simulink model "power_wind"  (R2014b)
settings: Solver=ode23tb  StartTime=0.0  StopTime=20  MaxStep=1/60  RelTol=1e-4  AbsTol=1e-3
InitFcn:
  | xInitial = init_power_wind_ig;
undefined symbols (not defined in the file): D1, D11, Delta
libraries: powerlib_meascontrol x45, powerlib x29, DRlib x3, factslib x1
(part 2 of 4)

== system power_wind/Wind Farm/Wind Turbine Protections/Protection System1/Decoding ==
  Code : Inport
  Constant : Constant  Value=pow2(0:-1:-9)
  Constant6 : Constant  Value=2
  Math Function : Math  Operator=rem  SaturateOnIntegerOverflow=on
  Product : Product  SaturateOnIntegerOverflow=on  InputSameDT=on  OutDataTypeStr=Inherit: Same as first input
  Rounding Function : Rounding
  Out : Outport
  wires:
  Math Function/1 -> Out/1
  Rounding Function/1 -> Math Function/1
  Constant6/1 -> Math Function/2
  Product/1 -> Rounding Function/1
  Code/1 -> Product/1
  Constant/1 -> Product/2

== system power_wind/Wind Farm/Wind Turbine Protections/Protection System1/Encoding ==
  In1 : Inport
  In2 : Inport  Port=2
  In3 : Inport  Port=3
  In4 : Inport  Port=4
  In5 : Inport  Port=5
  In6 : Inport  Port=6
  In7 : Inport  Port=7
  In8 : Inport  Port=8
  In9 : Inport  Port=9
  In10 : Inport  Port=10
  Constant12 : Constant  Value=pow2(0:1:9)
  Data Type Conversion : DataTypeConversion  SaturateOnIntegerOverflow=on  RndMeth=Zero
  Mux : Mux  Inputs=10
  Product : Product  SaturateOnIntegerOverflow=on  InputSameDT=on  OutDataTypeStr=Inherit: Same as first input
  Sum : Sum  Inputs=1  SaturateOnIntegerOverflow=on  InputSameDT=on  OutDataTypeStr=Inherit: Same as first input
  Code : Outport
  wires:
  Sum/1 -> Code/1
  Constant12/1 -> Product/2
  Product/1 -> Sum/1
  In1/1 -> Mux/1
  In10/1 -> Mux/10
  In9/1 -> Mux/9
  In8/1 -> Mux/8
  In7/1 -> Mux/7
  In6/1 -> Mux/6
  In5/1 -> Mux/5
  In4/1 -> Mux/4
  In3/1 -> Mux/3
  In2/1 -> Mux/2
  Mux/1 -> Data Type Conversion/1
  Data Type Conversion/1 -> Product/1

== system power_wind/Wind Farm/Wind Turbine Protections/Protection System1/Under//Over Speed Protection ==
  Speed : Inport  PortDimensions=1
  On Delay : powerlib_meascontrol/Logic/On Delay  DelayType=On delay  delay=Delay_Speed  ic=0  Ts=0
  On Delay1 : powerlib_meascontrol/Logic/On Delay  DelayType=On delay  delay=Delay_Speed  ic=0  Ts=0
  Relational Operator1 : RelationalOperator  Operator=>
  Relational Operator3 : RelationalOperator  Operator=<
  V1 max1 : Constant  Value=Min_Speed
  V1 max3 : Constant  Value=Max_Speed
  MinSpeed : Outport
  MaxSpeed : Outport  Port=2
  wires:
  On Delay1/1 -> MaxSpeed/1
  On Delay/1 -> MinSpeed/1
  Speed/1 -> Relational Operator1/1, Relational Operator3/1
  V1 max3/1 -> Relational Operator1/2
  V1 max1/1 -> Relational Operator3/2
  Relational Operator1/1 -> On Delay1/1
  Relational Operator3/1 -> On Delay/1

== system power_wind/Wind Farm/Wind Turbine Protections/Protection System2/AC Current Protection ==
  abc : Inport  PortDimensions=3
  Complex to Magnitude-Angle1 : ComplexToMagnitudeAngle  Output=Magnitude
  Current Measurement : Subsystem
  MinMax : MinMax  Function=max  ZeroCross=off  SaturateOnIntegerOverflow=on  InputSameDT=on
  Mux : Mux  Inputs=3
  On Delay : powerlib_meascontrol/Logic/On Delay  DelayType=On delay  delay=Delay_I1  ic=0  Ts=0
  On Delay1 : powerlib_meascontrol/Logic/On Delay  DelayType=On delay  delay=Delay_I2_I1  ic=0  Ts=0
  Relational Operator10 : RelationalOperator  Operator=>
  Relational Operator6 : RelationalOperator  Operator=>
  Relational Operator8 : RelationalOperator  Operator=>
  Selector : Selector  InputPortWidth=3
  Selector1 : Selector  InputPortWidth=3  Indices=2
  Selector2 : Selector  InputPortWidth=3  Indices=3
  V0/V1 max3 : Constant  Value=Max_I1
  V1 max : Constant  Value=Max_I2_I1
  V1 max2 : Constant  Value=Max_Iinst
  MaxIinst : Outport
  MaxI1 : Outport  Port=2
  MaxI2I1 : Outport  Port=3
  wires:
  abc/1 -> Current Measurement/1(abc), Selector/1, Selector1/1, Selector2/1
  Current Measurement/1(I1) -> Relational Operator6/1
  V0/V1 max3/1 -> Relational Operator6/2
  V1 max/1 -> Relational Operator8/2
  Current Measurement/2(I2/I1) -> Relational Operator8/1
  Relational Operator6/1 -> On Delay/1
  Relational Operator8/1 -> On Delay1/1
  On Delay/1 -> MaxI1/1
  On Delay1/1 -> MaxI2I1/1
  Relational Operator10/1 -> MaxIinst/1
  V1 max2/1 -> Relational Operator10/2
  Selector/1 -> Mux/1
  Selector2/1 -> Mux/3
  Selector1/1 -> Mux/2
  Mux/1 -> Complex to Magnitude-Angle1/1
  Complex to Magnitude-Angle1/1 -> MinMax/1
  MinMax/1 -> Relational Operator10/1

== system power_wind/Wind Farm/Wind Turbine Protections/Protection System2/AC Voltage Protection ==
  abc : Inport  PortDimensions=3
  On Delay : powerlib_meascontrol/Logic/On Delay  DelayType=On delay  delay=Delay_V1  ic=0  Ts=0
  On Delay1 : powerlib_meascontrol/Logic/On Delay  DelayType=On delay  delay=Delay_V1  ic=0  Ts=0
  On Delay2 : powerlib_meascontrol/Logic/On Delay  DelayType=On delay  delay=Delay_V2_V1  ic=0  Ts=0
  On Delay3 : powerlib_meascontrol/Logic/On Delay  DelayType=On delay  delay=Delay_V2_V1  ic=0  Ts=0
  Relational Operator6 : RelationalOperator  Operator=>
  Relational Operator7 : RelationalOperator  Operator=<
  Relational Operator8 : RelationalOperator  Operator=>
  Relational Operator9 : RelationalOperator  Operator=>
  V0/V1 max3 : Constant  Value=Max_V1
  V0/V1 max4 : Constant  Value=Min_V1
  V1 max : Constant  Value=Max_V2_V1
  V1 max1 : Constant  Value=Max_V0_V1
  Voltage Measurement : Subsystem
  MinV1 : Outport
  MaxV1 : Outport  Port=2
  MaxV2V1 : Outport  Port=3
  MaxV0V1 : Outport  Port=4
  wires:
  On Delay3/1 -> MaxV0V1/1
  On Delay2/1 -> MaxV2V1/1
  On Delay/1 -> MinV1/1
  On Delay1/1 -> MaxV1/1
  Relational Operator9/1 -> On Delay3/1
  Relational Operator8/1 -> On Delay2/1
  Relational Operator7/1 -> On Delay/1
  Relational Operator6/1 -> On Delay1/1
  Voltage Measurement/3(V0/V1) -> Relational Operator9/1
  V1 max1/1 -> Relational Operator9/2
  Voltage Measurement/2(V2/V1) -> Relational Operator8/1
  V1 max/1 -> Relational Operator8/2
  V0/V1 max4/1 -> Relational Operator7/2
  V0/V1 max3/1 -> Relational Operator6/2
  Voltage Measurement/1(V1) -> Relational Operator7/1, Relational Operator6/1
  abc/1 -> Voltage Measurement/1(abc)

== system power_wind/Wind Farm/Wind Turbine Protections/Protection System2/DC Voltage Protection ==
  Vdc : Inport
  On Delay : powerlib_meascontrol/Logic/On Delay  DelayType=On delay  delay=Delay_Vdc  ic=0  Ts=0
  Relational Operator1 : RelationalOperator  Operator=>
  V1 max3 : Constant  Value=Max_Vdc
  MaxVdc : Outport
  wires:
  Vdc/1 -> Relational Operator1/1
  V1 max3/1 -> Relational Operator1/2
  Relational Operator1/1 -> On Delay/1
  On Delay/1 -> MaxVdc/1

== system power_wind/Wind Farm/Wind Turbine Protections/Protection System2/Decoding ==
  Code : Inport
  Constant : Constant  Value=pow2(0:-1:-9)
  Constant6 : Constant  Value=2
  Math Function : Math  Operator=rem  SaturateOnIntegerOverflow=on
  Product : Product  SaturateOnIntegerOverflow=on  InputSameDT=on  OutDataTypeStr=Inherit: Same as first input
  Rounding Function : Rounding
  Out : Outport
  wires:
  Constant/1 -> Product/2
  Code/1 -> Product/1
  Product/1 -> Rounding Function/1
  Constant6/1 -> Math Function/2
  Rounding Function/1 -> Math Function/1
  Math Function/1 -> Out/1

== system power_wind/Wind Farm/Wind Turbine Protections/Protection System2/Encoding ==
  In1 : Inport
  In2 : Inport  Port=2
  In3 : Inport  Port=3
  In4 : Inport  Port=4
  In5 : Inport  Port=5
  In6 : Inport  Port=6
  In7 : Inport  Port=7
  In8 : Inport  Port=8
  In9 : Inport  Port=9
  In10 : Inport  Port=10
  Constant12 : Constant  Value=pow2(0:1:9)
  Data Type Conversion : DataTypeConversion  SaturateOnIntegerOverflow=on  RndMeth=Zero
  Mux : Mux  Inputs=10
  Product : Product  SaturateOnIntegerOverflow=on  InputSameDT=on  OutDataTypeStr=Inherit: Same as first input
  Sum : Sum  Inputs=1  SaturateOnIntegerOverflow=on  InputSameDT=on  OutDataTypeStr=Inherit: Same as first input
  Code : Outport
  wires:
  Data Type Conversion/1 -> Product/1
  Mux/1 -> Data Type Conversion/1
  In2/1 -> Mux/2
  In3/1 -> Mux/3
  In4/1 -> Mux/4
  In5/1 -> Mux/5
  In6/1 -> Mux/6
  In7/1 -> Mux/7
  In8/1 -> Mux/8
  In9/1 -> Mux/9
  In10/1 -> Mux/10
  In1/1 -> Mux/1
  Product/1 -> Sum/1
  Constant12/1 -> Product/2
  Sum/1 -> Code/1

== system power_wind/Wind Farm/Wind Turbine Protections/Protection System2/Under//Over Speed Protection ==
  Speed : Inport  PortDimensions=1
  On Delay : powerlib_meascontrol/Logic/On Delay  DelayType=On delay  delay=Delay_Speed  ic=0  Ts=0
  On Delay1 : powerlib_meascontrol/Logic/On Delay  DelayType=On delay  delay=Delay_Speed  ic=0  Ts=0
  Relational Operator1 : RelationalOperator  Operator=>
  Relational Operator3 : RelationalOperator  Operator=<
  V1 max1 : Constant  Value=Min_Speed
  V1 max3 : Constant  Value=Max_Speed
  MinSpeed : Outport
  MaxSpeed : Outport  Port=2
  wires:
  Relational Operator3/1 -> On Delay/1
  Relational Operator1/1 -> On Delay1/1
  V1 max1/1 -> Relational Operator3/2
  V1 max3/1 -> Relational Operator1/2
  Speed/1 -> Relational Operator3/1, Relational Operator1/1
  On Delay/1 -> MinSpeed/1
  On Delay1/1 -> MaxSpeed/1

== system power_wind/Wind Farm/Wind Turbine Protections/Protection System3/AC Current Protection ==
  abc : Inport  PortDimensions=3
  Complex to Magnitude-Angle1 : ComplexToMagnitudeAngle  Output=Magnitude
  Current Measurement : Subsystem
  MinMax : MinMax  Function=max  ZeroCross=off  SaturateOnIntegerOverflow=on  InputSameDT=on
  Mux : Mux  Inputs=3
  On Delay : powerlib_meascontrol/Logic/On Delay  DelayType=On delay  delay=Delay_I1  ic=0  Ts=0
  On Delay1 : powerlib_meascontrol/Logic/On Delay  DelayType=On delay  delay=Delay_I2_I1  ic=0  Ts=0
  Relational Operator10 : RelationalOperator  Operator=>
  Relational Operator6 : RelationalOperator  Operator=>
  Relational Operator8 : RelationalOperator  Operator=>
  Selector : Selector  InputPortWidth=3
  Selector1 : Selector  InputPortWidth=3  Indices=2
  Selector2 : Selector  InputPortWidth=3  Indices=3
  V0/V1 max3 : Constant  Value=Max_I1
  V1 max : Constant  Value=Max_I2_I1
  V1 max2 : Constant  Value=Max_Iinst
  MaxIinst : Outport
  MaxI1 : Outport  Port=2
  MaxI2I1 : Outport  Port=3
  wires:
  MinMax/1 -> Relational Operator10/1
  Complex to Magnitude-Angle1/1 -> MinMax/1
  Mux/1 -> Complex to Magnitude-Angle1/1
  Selector1/1 -> Mux/2
  Selector2/1 -> Mux/3
  Selector/1 -> Mux/1
  V1 max2/1 -> Relational Operator10/2
  Relational Operator10/1 -> MaxIinst/1
  On Delay1/1 -> MaxI2I1/1
  On Delay/1 -> MaxI1/1
  Relational Operator8/1 -> On Delay1/1
  Relational Operator6/1 -> On Delay/1
  Current Measurement/2(I2/I1) -> Relational Operator8/1
  V1 max/1 -> Relational Operator8/2
  V0/V1 max3/1 -> Relational Operator6/2
  Current Measurement/1(I1) -> Relational Operator6/1
  abc/1 -> Selector2/1, Selector1/1, Selector/1, Current Measurement/1(abc)

== system power_wind/Wind Farm/Wind Turbine Protections/Protection System3/AC Voltage Protection ==
  abc : Inport  PortDimensions=3
  On Delay : powerlib_meascontrol/Logic/On Delay  DelayType=On delay  delay=Delay_V1  ic=0  Ts=0
  On Delay1 : powerlib_meascontrol/Logic/On Delay  DelayType=On delay  delay=Delay_V1  ic=0  Ts=0
  On Delay2 : powerlib_meascontrol/Logic/On Delay  DelayType=On delay  delay=Delay_V2_V1  ic=0  Ts=0
  On Delay3 : powerlib_meascontrol/Logic/On Delay  DelayType=On delay  delay=Delay_V2_V1  ic=0  Ts=0
  Relational Operator6 : RelationalOperator  Operator=>
  Relational Operator7 : RelationalOperator  Operator=<
  Relational Operator8 : RelationalOperator  Operator=>
  Relational Operator9 : RelationalOperator  Operator=>
  V0/V1 max3 : Constant  Value=Max_V1
  V0/V1 max4 : Constant  Value=Min_V1
  V1 max : Constant  Value=Max_V2_V1
  V1 max1 : Constant  Value=Max_V0_V1
  Voltage Measurement : Subsystem
  MinV1 : Outport
  MaxV1 : Outport  Port=2
  MaxV2V1 : Outport  Port=3
  MaxV0V1 : Outport  Port=4
  wires:
  abc/1 -> Voltage Measurement/1(abc)
  Voltage Measurement/1(V1) -> Relational Operator6/1, Relational Operator7/1
  V0/V1 max3/1 -> Relational Operator6/2
  V0/V1 max4/1 -> Relational Operator7/2
  V1 max/1 -> Relational Operator8/2
  Voltage Measurement/2(V2/V1) -> Relational Operator8/1
  V1 max1/1 -> Relational Operator9/2
  Voltage Measurement/3(V0/V1) -> Relational Operator9/1
  Relational Operator6/1 -> On Delay1/1
  Relational Operator7/1 -> On Delay/1
  Relational Operator8/1 -> On Delay2/1
  Relational Operator9/1 -> On Delay3/1
  On Delay1/1 -> MaxV1/1
  On Delay/1 -> MinV1/1
  On Delay2/1 -> MaxV2V1/1
  On Delay3/1 -> MaxV0V1/1

== system power_wind/Wind Farm/Wind Turbine Protections/Protection System3/DC Voltage Protection ==
  Vdc : Inport
  On Delay : powerlib_meascontrol/Logic/On Delay  DelayType=On delay  delay=Delay_Vdc  ic=0  Ts=0
  Relational Operator1 : RelationalOperator  Operator=>
  V1 max3 : Constant  Value=Max_Vdc
  MaxVdc : Outport
  wires:
  On Delay/1 -> MaxVdc/1
  Relational Operator1/1 -> On Delay/1
  V1 max3/1 -> Relational Operator1/2
  Vdc/1 -> Relational Operator1/1

== system power_wind/Wind Farm/Wind Turbine Protections/Protection System3/Decoding ==
  Code : Inport
  Constant : Constant  Value=pow2(0:-1:-9)
  Constant6 : Constant  Value=2
  Math Function : Math  Operator=rem  SaturateOnIntegerOverflow=on
  Product : Product  SaturateOnIntegerOverflow=on  InputSameDT=on  OutDataTypeStr=Inherit: Same as first input
  Rounding Function : Rounding
  Out : Outport
  wires:
  Math Function/1 -> Out/1
  Rounding Function/1 -> Math Function/1
  Constant6/1 -> Math Function/2
  Product/1 -> Rounding Function/1
  Code/1 -> Product/1
  Constant/1 -> Product/2

== system power_wind/Wind Farm/Wind Turbine Protections/Protection System3/Encoding ==
  In1 : Inport
  In2 : Inport  Port=2
  In3 : Inport  Port=3
  In4 : Inport  Port=4
  In5 : Inport  Port=5
  In6 : Inport  Port=6
  In7 : Inport  Port=7
  In8 : Inport  Port=8
  In9 : Inport  Port=9
  In10 : Inport  Port=10
  Constant12 : Constant  Value=pow2(0:1:9)
  Data Type Conversion : DataTypeConversion  SaturateOnIntegerOverflow=on  RndMeth=Zero
  Mux : Mux  Inputs=10
  Product : Product  SaturateOnIntegerOverflow=on  InputSameDT=on  OutDataTypeStr=Inherit: Same as first input
  Sum : Sum  Inputs=1  SaturateOnIntegerOverflow=on  InputSameDT=on  OutDataTypeStr=Inherit: Same as first input
  Code : Outport
  wires:
  Sum/1 -> Code/1
  Constant12/1 -> Product/2
  Product/1 -> Sum/1
  In1/1 -> Mux/1
  In10/1 -> Mux/10
  In9/1 -> Mux/9
  In8/1 -> Mux/8
  In7/1 -> Mux/7
  In6/1 -> Mux/6
  In5/1 -> Mux/5
  In4/1 -> Mux/4
  In3/1 -> Mux/3
  In2/1 -> Mux/2
  Mux/1 -> Data Type Conversion/1
  Data Type Conversion/1 -> Product/1

== system power_wind/Wind Farm/Wind Turbine Protections/Protection System3/Under//Over Speed Protection ==
  Speed : Inport  PortDimensions=1
  On Delay : powerlib_meascontrol/Logic/On Delay  DelayType=On delay  delay=Delay_Speed  ic=0  Ts=0
  On Delay1 : powerlib_meascontrol/Logic/On Delay  DelayType=On delay  delay=Delay_Speed  ic=0  Ts=0
  Relational Operator1 : RelationalOperator  Operator=>
  Relational Operator3 : RelationalOperator  Operator=<
  V1 max1 : Constant  Value=Min_Speed
  V1 max3 : Constant  Value=Max_Speed
  MinSpeed : Outport
  MaxSpeed : Outport  Port=2
  wires:
  On Delay1/1 -> MaxSpeed/1
  On Delay/1 -> MinSpeed/1
  Speed/1 -> Relational Operator1/1, Relational Operator3/1
  V1 max3/1 -> Relational Operator1/2
  V1 max1/1 -> Relational Operator3/2
  Relational Operator1/1 -> On Delay1/1
  Relational Operator3/1 -> On Delay/1

== system power_wind/Wind Farm/Wind Turbine Protections/Protection System1/AC Current Protection/Current Measurement ==
  abc : Inport  PortDimensions=3
  Gain1 : Gain  Gain=[1 a a2]  SaturateOnIntegerOverflow=on  OutDataTypeStr=Inherit: Same as input  ParamDataTypeStr=Inherit: Same as input
  Gain2 : Gain  Gain=[1 a2 a]  SaturateOnIntegerOverflow=on  OutDataTypeStr=Inherit: Same as input  ParamDataTypeStr=Inherit: Same as input
  Gain3 : Gain  Gain=1/3  SaturateOnIntegerOverflow=on  OutDataTypeStr=Inherit: Same as input  ParamDataTypeStr=Inherit: Same as input
  Gain4 : Gain  Gain=1/3  SaturateOnIntegerOverflow=on  OutDataTypeStr=Inherit: Same as input  ParamDataTypeStr=Inherit: Same as input
  Mux : Mux  Inputs=3
  Product : Product  Inputs=/*  SaturateOnIntegerOverflow=on  OutDataTypeStr=Inherit: Same as first input
  Saturation : Saturate  UpperLimit=1e6  LowerLimit=1e-6
  Selector : Selector  InputPortWidth=3
  Selector1 : Selector  InputPortWidth=3  Indices=2
  Selector2 : Selector  InputPortWidth=3  Indices=3
  Sum : Sum  Inputs=1  SaturateOnIntegerOverflow=on  InputSameDT=on  OutDataTypeStr=Inherit: Same as first input
  Sum1 : Sum  Inputs=1  SaturateOnIntegerOverflow=on  InputSameDT=on  OutDataTypeStr=Inherit: Same as first input
  magnitude : Subsystem
  magnitude1 : Subsystem
  I1 : Outport
  I2/I1 : Outport  Port=2
  wires:
  magnitude/1(Out1) -> I1/1, Saturation/1
  magnitude1/1(Out1) -> Product/2
  Product/1 -> I2/I1/1
  Saturation/1 -> Product/1
  Gain4/1 -> magnitude1/1(In1)
  Gain3/1 -> magnitude/1(In1)
  Mux/1 -> Gain2/1, Gain1/1
  abc/1 -> Selector/1, Selector1/1, Selector2/1
  Gain2/1 -> Sum1/1
  Sum1/1 -> Gain4/1
  Gain1/1 -> Sum/1
  Sum/1 -> Gain3/1
  Selector/1 -> Mux/1
  Selector1/1 -> Mux/2
  Selector2/1 -> Mux/3

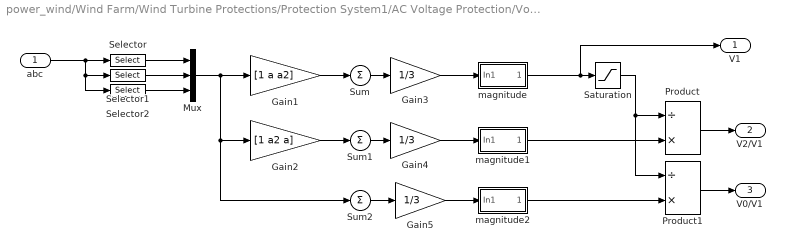
== system power_wind/Wind Farm/Wind Turbine Protections/Protection System1/AC Voltage Protection/Voltage Measurement ==
  abc : Inport  PortDimensions=3
  Gain1 : Gain  Gain=[1 a a2]  SaturateOnIntegerOverflow=on  OutDataTypeStr=Inherit: Same as input  ParamDataTypeStr=Inherit: Same as input
  Gain2 : Gain  Gain=[1 a2 a]  SaturateOnIntegerOverflow=on  OutDataTypeStr=Inherit: Same as input  ParamDataTypeStr=Inherit: Same as input
  Gain3 : Gain  Gain=1/3  SaturateOnIntegerOverflow=on  OutDataTypeStr=Inherit: Same as input  ParamDataTypeStr=Inherit: Same as input
  Gain4 : Gain  Gain=1/3  SaturateOnIntegerOverflow=on  OutDataTypeStr=Inherit: Same as input  ParamDataTypeStr=Inherit: Same as input
  Gain5 : Gain  Gain=1/3  SaturateOnIntegerOverflow=on  OutDataTypeStr=Inherit: Same as input  ParamDataTypeStr=Inherit: Same as input
  Mux : Mux  Inputs=3
  Product : Product  Inputs=/*  SaturateOnIntegerOverflow=on  OutDataTypeStr=Inherit: Same as first input
  Product1 : Product  Inputs=/*  SaturateOnIntegerOverflow=on  OutDataTypeStr=Inherit: Same as first input
  Saturation : Saturate  UpperLimit=1e6  LowerLimit=1e-6
  Selector : Selector  InputPortWidth=3
  Selector1 : Selector  InputPortWidth=3  Indices=2
  Selector2 : Selector  InputPortWidth=3  Indices=3
  Sum : Sum  Inputs=1  SaturateOnIntegerOverflow=on  InputSameDT=on  OutDataTypeStr=Inherit: Same as first input
  Sum1 : Sum  Inputs=1  SaturateOnIntegerOverflow=on  InputSameDT=on  OutDataTypeStr=Inherit: Same as first input
  Sum2 : Sum  Inputs=1  SaturateOnIntegerOverflow=on  InputSameDT=on  OutDataTypeStr=Inherit: Same as first input
  magnitude : Subsystem
  magnitude1 : Subsystem
  magnitude2 : Subsystem
  V1 : Outport
  V2/V1 : Outport  Port=2
  V0/V1 : Outport  Port=3
  wires:
  magnitude2/1(Out1) -> Product1/2
  magnitude1/1(Out1) -> Product/2
  magnitude/1(Out1) -> Saturation/1, V1/1
  Sum/1 -> Gain3/1
  Gain1/1 -> Sum/1
  Sum1/1 -> Gain4/1
  Gain2/1 -> Sum1/1
  Sum2/1 -> Gain5/1
  Mux/1 -> Gain1/1, Gain2/1, Sum2/1
  Gain3/1 -> magnitude/1(In1)
  Gain4/1 -> magnitude1/1(In1)
  Saturation/1 -> Product/1, Product1/1
  Gain5/1 -> magnitude2/1(In1)
  Product/1 -> V2/V1/1
  Product1/1 -> V0/V1/1
  abc/1 -> Selector/1, Selector1/1, Selector2/1
  Selector/1 -> Mux/1
  Selector1/1 -> Mux/2
  Selector2/1 -> Mux/3

== system power_wind/Wind Farm/Wind Turbine Protections/Protection System2/AC Current Protection/Current Measurement ==
  abc : Inport  PortDimensions=3
  Gain1 : Gain  Gain=[1 a a2]  SaturateOnIntegerOverflow=on  OutDataTypeStr=Inherit: Same as input  ParamDataTypeStr=Inherit: Same as input
  Gain2 : Gain  Gain=[1 a2 a]  SaturateOnIntegerOverflow=on  OutDataTypeStr=Inherit: Same as input  ParamDataTypeStr=Inherit: Same as input
  Gain3 : Gain  Gain=1/3  SaturateOnIntegerOverflow=on  OutDataTypeStr=Inherit: Same as input  ParamDataTypeStr=Inherit: Same as input
  Gain4 : Gain  Gain=1/3  SaturateOnIntegerOverflow=on  OutDataTypeStr=Inherit: Same as input  ParamDataTypeStr=Inherit: Same as input
  Mux : Mux  Inputs=3
  Product : Product  Inputs=/*  SaturateOnIntegerOverflow=on  OutDataTypeStr=Inherit: Same as first input
  Saturation : Saturate  UpperLimit=1e6  LowerLimit=1e-6
  Selector : Selector  InputPortWidth=3
  Selector1 : Selector  InputPortWidth=3  Indices=2
  Selector2 : Selector  InputPortWidth=3  Indices=3
  Sum : Sum  Inputs=1  SaturateOnIntegerOverflow=on  InputSameDT=on  OutDataTypeStr=Inherit: Same as first input
  Sum1 : Sum  Inputs=1  SaturateOnIntegerOverflow=on  InputSameDT=on  OutDataTypeStr=Inherit: Same as first input
  magnitude : Subsystem
  magnitude1 : Subsystem
  I1 : Outport
  I2/I1 : Outport  Port=2
  wires:
  Selector2/1 -> Mux/3
  Selector1/1 -> Mux/2
  Selector/1 -> Mux/1
  Sum/1 -> Gain3/1
  Gain1/1 -> Sum/1
  Sum1/1 -> Gain4/1
  Gain2/1 -> Sum1/1
  abc/1 -> Selector2/1, Selector1/1, Selector/1
  Mux/1 -> Gain1/1, Gain2/1
  Gain3/1 -> magnitude/1(In1)
  Gain4/1 -> magnitude1/1(In1)
  Saturation/1 -> Product/1
  Product/1 -> I2/I1/1
  magnitude1/1(Out1) -> Product/2
  magnitude/1(Out1) -> Saturation/1, I1/1

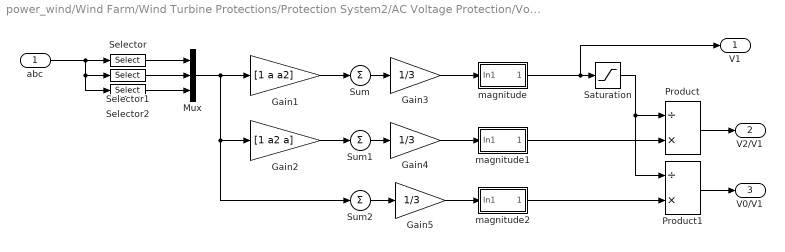
== system power_wind/Wind Farm/Wind Turbine Protections/Protection System2/AC Voltage Protection/Voltage Measurement ==
  abc : Inport  PortDimensions=3
  Gain1 : Gain  Gain=[1 a a2]  SaturateOnIntegerOverflow=on  OutDataTypeStr=Inherit: Same as input  ParamDataTypeStr=Inherit: Same as input
  Gain2 : Gain  Gain=[1 a2 a]  SaturateOnIntegerOverflow=on  OutDataTypeStr=Inherit: Same as input  ParamDataTypeStr=Inherit: Same as input
  Gain3 : Gain  Gain=1/3  SaturateOnIntegerOverflow=on  OutDataTypeStr=Inherit: Same as input  ParamDataTypeStr=Inherit: Same as input
  Gain4 : Gain  Gain=1/3  SaturateOnIntegerOverflow=on  OutDataTypeStr=Inherit: Same as input  ParamDataTypeStr=Inherit: Same as input
  Gain5 : Gain  Gain=1/3  SaturateOnIntegerOverflow=on  OutDataTypeStr=Inherit: Same as input  ParamDataTypeStr=Inherit: Same as input
  Mux : Mux  Inputs=3
  Product : Product  Inputs=/*  SaturateOnIntegerOverflow=on  OutDataTypeStr=Inherit: Same as first input
  Product1 : Product  Inputs=/*  SaturateOnIntegerOverflow=on  OutDataTypeStr=Inherit: Same as first input
  Saturation : Saturate  UpperLimit=1e6  LowerLimit=1e-6
  Selector : Selector  InputPortWidth=3
  Selector1 : Selector  InputPortWidth=3  Indices=2
  Selector2 : Selector  InputPortWidth=3  Indices=3
  Sum : Sum  Inputs=1  SaturateOnIntegerOverflow=on  InputSameDT=on  OutDataTypeStr=Inherit: Same as first input
  Sum1 : Sum  Inputs=1  SaturateOnIntegerOverflow=on  InputSameDT=on  OutDataTypeStr=Inherit: Same as first input
  Sum2 : Sum  Inputs=1  SaturateOnIntegerOverflow=on  InputSameDT=on  OutDataTypeStr=Inherit: Same as first input
  magnitude : Subsystem
  magnitude1 : Subsystem
  magnitude2 : Subsystem
  V1 : Outport
  V2/V1 : Outport  Port=2
  V0/V1 : Outport  Port=3
  wires:
  Selector2/1 -> Mux/3
  Selector1/1 -> Mux/2
  Selector/1 -> Mux/1
  abc/1 -> Selector2/1, Selector1/1, Selector/1
  Product1/1 -> V0/V1/1
  Product/1 -> V2/V1/1
  Gain5/1 -> magnitude2/1(In1)
  Saturation/1 -> Product1/1, Product/1
  Gain4/1 -> magnitude1/1(In1)
  Gain3/1 -> magnitude/1(In1)
  Mux/1 -> Sum2/1, Gain2/1, Gain1/1
  Sum2/1 -> Gain5/1
  Gain2/1 -> Sum1/1
  Sum1/1 -> Gain4/1
  Gain1/1 -> Sum/1
  Sum/1 -> Gain3/1
  magnitude/1(Out1) -> V1/1, Saturation/1
  magnitude1/1(Out1) -> Product/2
  magnitude2/1(Out1) -> Product1/2

== system power_wind/Wind Farm/Wind Turbine Protections/Protection System3/AC Current Protection/Current Measurement ==
  abc : Inport  PortDimensions=3
  Gain1 : Gain  Gain=[1 a a2]  SaturateOnIntegerOverflow=on  OutDataTypeStr=Inherit: Same as input  ParamDataTypeStr=Inherit: Same as input
  Gain2 : Gain  Gain=[1 a2 a]  SaturateOnIntegerOverflow=on  OutDataTypeStr=Inherit: Same as input  ParamDataTypeStr=Inherit: Same as input
  Gain3 : Gain  Gain=1/3  SaturateOnIntegerOverflow=on  OutDataTypeStr=Inherit: Same as input  ParamDataTypeStr=Inherit: Same as input
  Gain4 : Gain  Gain=1/3  SaturateOnIntegerOverflow=on  OutDataTypeStr=Inherit: Same as input  ParamDataTypeStr=Inherit: Same as input
  Mux : Mux  Inputs=3
  Product : Product  Inputs=/*  SaturateOnIntegerOverflow=on  OutDataTypeStr=Inherit: Same as first input
  Saturation : Saturate  UpperLimit=1e6  LowerLimit=1e-6
  Selector : Selector  InputPortWidth=3
  Selector1 : Selector  InputPortWidth=3  Indices=2
  Selector2 : Selector  InputPortWidth=3  Indices=3
  Sum : Sum  Inputs=1  SaturateOnIntegerOverflow=on  InputSameDT=on  OutDataTypeStr=Inherit: Same as first input
  Sum1 : Sum  Inputs=1  SaturateOnIntegerOverflow=on  InputSameDT=on  OutDataTypeStr=Inherit: Same as first input
  magnitude : Subsystem
  magnitude1 : Subsystem
  I1 : Outport
  I2/I1 : Outport  Port=2
  wires:
  magnitude/1(Out1) -> I1/1, Saturation/1
  magnitude1/1(Out1) -> Product/2
  Product/1 -> I2/I1/1
  Saturation/1 -> Product/1
  Gain4/1 -> magnitude1/1(In1)
  Gain3/1 -> magnitude/1(In1)
  Mux/1 -> Gain2/1, Gain1/1
  abc/1 -> Selector/1, Selector1/1, Selector2/1
  Gain2/1 -> Sum1/1
  Sum1/1 -> Gain4/1
  Gain1/1 -> Sum/1
  Sum/1 -> Gain3/1
  Selector/1 -> Mux/1
  Selector1/1 -> Mux/2
  Selector2/1 -> Mux/3

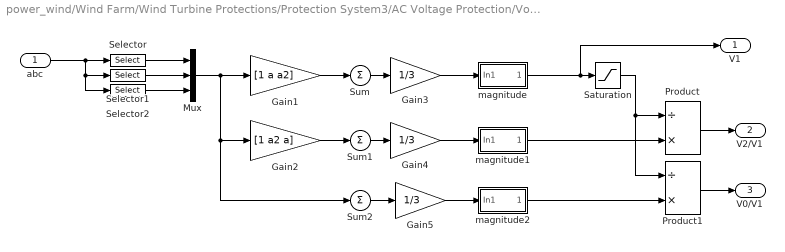
== system power_wind/Wind Farm/Wind Turbine Protections/Protection System3/AC Voltage Protection/Voltage Measurement ==
  abc : Inport  PortDimensions=3
  Gain1 : Gain  Gain=[1 a a2]  SaturateOnIntegerOverflow=on  OutDataTypeStr=Inherit: Same as input  ParamDataTypeStr=Inherit: Same as input
  Gain2 : Gain  Gain=[1 a2 a]  SaturateOnIntegerOverflow=on  OutDataTypeStr=Inherit: Same as input  ParamDataTypeStr=Inherit: Same as input
  Gain3 : Gain  Gain=1/3  SaturateOnIntegerOverflow=on  OutDataTypeStr=Inherit: Same as input  ParamDataTypeStr=Inherit: Same as input
  Gain4 : Gain  Gain=1/3  SaturateOnIntegerOverflow=on  OutDataTypeStr=Inherit: Same as input  ParamDataTypeStr=Inherit: Same as input
  Gain5 : Gain  Gain=1/3  SaturateOnIntegerOverflow=on  OutDataTypeStr=Inherit: Same as input  ParamDataTypeStr=Inherit: Same as input
  Mux : Mux  Inputs=3
  Product : Product  Inputs=/*  SaturateOnIntegerOverflow=on  OutDataTypeStr=Inherit: Same as first input
  Product1 : Product  Inputs=/*  SaturateOnIntegerOverflow=on  OutDataTypeStr=Inherit: Same as first input
  Saturation : Saturate  UpperLimit=1e6  LowerLimit=1e-6
  Selector : Selector  InputPortWidth=3
  Selector1 : Selector  InputPortWidth=3  Indices=2
  Selector2 : Selector  InputPortWidth=3  Indices=3
  Sum : Sum  Inputs=1  SaturateOnIntegerOverflow=on  InputSameDT=on  OutDataTypeStr=Inherit: Same as first input
  Sum1 : Sum  Inputs=1  SaturateOnIntegerOverflow=on  InputSameDT=on  OutDataTypeStr=Inherit: Same as first input
  Sum2 : Sum  Inputs=1  SaturateOnIntegerOverflow=on  InputSameDT=on  OutDataTypeStr=Inherit: Same as first input
  magnitude : Subsystem
  magnitude1 : Subsystem
  magnitude2 : Subsystem
  V1 : Outport
  V2/V1 : Outport  Port=2
  V0/V1 : Outport  Port=3
  wires:
  magnitude2/1(Out1) -> Product1/2
  magnitude1/1(Out1) -> Product/2
  magnitude/1(Out1) -> Saturation/1, V1/1
  Sum/1 -> Gain3/1
  Gain1/1 -> Sum/1
  Sum1/1 -> Gain4/1
  Gain2/1 -> Sum1/1
  Sum2/1 -> Gain5/1
  Mux/1 -> Gain1/1, Gain2/1, Sum2/1
  Gain3/1 -> magnitude/1(In1)
  Gain4/1 -> magnitude1/1(In1)
  Saturation/1 -> Product/1, Product1/1
  Gain5/1 -> magnitude2/1(In1)
  Product/1 -> V2/V1/1
  Product1/1 -> V0/V1/1
  abc/1 -> Selector/1, Selector1/1, Selector2/1
  Selector/1 -> Mux/1
  Selector1/1 -> Mux/2
  Selector2/1 -> Mux/3

== system power_wind/Wind Farm/Wind Turbine Protections/Protection System1/AC Current Protection/Current Measurement/magnitude ==
  In1 : Inport
  Complex to Real-Imag : ComplexToRealImag
  Fourier1 : Subsystem  mask(Fourier analyser){f1=Freq, n=0}
      mask prompts: f1 "Fundamental frequency f1 (Hz):"; n "Harmonic n (0=DC; 1=fundamental; 2=2nd harm;  ...) :"
      mask help: The Fourier block performs a Fourier analysis of the input signal over a running window of one cycle of the fundamental frequency. First and second outputs return respectively the magnitude and phase (degrees) of the harmonic component specified.
      mask init:
      | k=2-(n==0);
      mask Help: helpview(psbhelp)
  Fourier2 : Subsystem  mask(Fourier analyser){f1=Freq, n=0}
      mask prompts: f1 "Fundamental frequency f1 (Hz):"; n "Harmonic n (0=DC; 1=fundamental; 2=2nd harm;  ...) :"
      mask help: The Fourier block performs a Fourier analysis of the input signal over a running window of one cycle of the fundamental frequency. First and second outputs return respectively the magnitude and phase (degrees) of the harmonic component specified.
      mask init:
      | k=2-(n==0);
      mask Help: helpview(psbhelp)
  Math Function : Math  Operator=hypot  SaturateOnIntegerOverflow=on
  Terminator : Terminator
  Terminator1 : Terminator
  Out1 : Outport
  wires:
  In1/1 -> Complex to Real-Imag/1
  Math Function/1 -> Out1/1
  Fourier2/1(magnitude) -> Math Function/2
  Fourier1/1(magnitude) -> Math Function/1
  Fourier2/2(angle) -> Terminator1/1
  Fourier1/2(angle) -> Terminator/1
  Complex to Real-Imag/2 -> Fourier2/1(signal)
  Complex to Real-Imag/1 -> Fourier1/1(signal)

== system power_wind/Wind Farm/Wind Turbine Protections/Protection System1/AC Current Protection/Current Measurement/magnitude1 ==
  In1 : Inport
  Complex to Real-Imag : ComplexToRealImag
  Fourier1 : Subsystem  mask(Fourier analyser){f1=Freq, n=0}
      mask prompts: f1 "Fundamental frequency f1 (Hz):"; n "Harmonic n (0=DC; 1=fundamental; 2=2nd harm;  ...) :"
      mask help: The Fourier block performs a Fourier analysis of the input signal over a running window of one cycle of the fundamental frequency. First and second outputs return respectively the magnitude and phase (degrees) of the harmonic component specified.
      mask init:
      | k=2-(n==0);
      mask Help: helpview(psbhelp)
  Fourier2 : Subsystem  mask(Fourier analyser){f1=Freq, n=0}
      mask prompts: f1 "Fundamental frequency f1 (Hz):"; n "Harmonic n (0=DC; 1=fundamental; 2=2nd harm;  ...) :"
      mask help: The Fourier block performs a Fourier analysis of the input signal over a running window of one cycle of the fundamental frequency. First and second outputs return respectively the magnitude and phase (degrees) of the harmonic component specified.
      mask init:
      | k=2-(n==0);
      mask Help: helpview(psbhelp)
  Math Function : Math  Operator=hypot  SaturateOnIntegerOverflow=on
  Terminator : Terminator
  Terminator1 : Terminator
  Out1 : Outport
  wires:
  Complex to Real-Imag/1 -> Fourier1/1(signal)
  Complex to Real-Imag/2 -> Fourier2/1(signal)
  Fourier1/2(angle) -> Terminator/1
  Fourier2/2(angle) -> Terminator1/1
  Fourier1/1(magnitude) -> Math Function/1
  Fourier2/1(magnitude) -> Math Function/2
  Math Function/1 -> Out1/1
  In1/1 -> Complex to Real-Imag/1

== system power_wind/Wind Farm/Wind Turbine Protections/Protection System1/AC Voltage Protection/Voltage Measurement/magnitude ==
  In1 : Inport
  Complex to Real-Imag : ComplexToRealImag
  Fourier1 : Subsystem  mask(Fourier analyser){f1=Freq, n=0}
      mask prompts: f1 "Fundamental frequency f1 (Hz):"; n "Harmonic n (0=DC; 1=fundamental; 2=2nd harm;  ...) :"
      mask help: The Fourier block performs a Fourier analysis of the input signal over a running window of one cycle of the fundamental frequency. First and second outputs return respectively the magnitude and phase (degrees) of the harmonic component specified.
      mask init:
      | k=2-(n==0);
      mask Help: helpview(psbhelp)
  Fourier2 : Subsystem  mask(Fourier analyser){f1=Freq, n=0}
      mask prompts: f1 "Fundamental frequency f1 (Hz):"; n "Harmonic n (0=DC; 1=fundamental; 2=2nd harm;  ...) :"
      mask help: The Fourier block performs a Fourier analysis of the input signal over a running window of one cycle of the fundamental frequency. First and second outputs return respectively the magnitude and phase (degrees) of the harmonic component specified.
      mask init:
      | k=2-(n==0);
      mask Help: helpview(psbhelp)
  Math Function : Math  Operator=hypot  SaturateOnIntegerOverflow=on
  Terminator : Terminator
  Terminator1 : Terminator
  Out1 : Outport
  wires:
  In1/1 -> Complex to Real-Imag/1
  Math Function/1 -> Out1/1
  Fourier2/1(magnitude) -> Math Function/2
  Fourier1/1(magnitude) -> Math Function/1
  Fourier2/2(angle) -> Terminator1/1
  Fourier1/2(angle) -> Terminator/1
  Complex to Real-Imag/2 -> Fourier2/1(signal)
  Complex to Real-Imag/1 -> Fourier1/1(signal)

== system power_wind/Wind Farm/Wind Turbine Protections/Protection System1/AC Voltage Protection/Voltage Measurement/magnitude1 ==
  In1 : Inport
  Complex to Real-Imag : ComplexToRealImag
  Fourier1 : Subsystem  mask(Fourier analyser){f1=Freq, n=0}
      mask prompts: f1 "Fundamental frequency f1 (Hz):"; n "Harmonic n (0=DC; 1=fundamental; 2=2nd harm;  ...) :"
      mask help: The Fourier block performs a Fourier analysis of the input signal over a running window of one cycle of the fundamental frequency. First and second outputs return respectively the magnitude and phase (degrees) of the harmonic component specified.
      mask init:
      | k=2-(n==0);
      mask Help: helpview(psbhelp)
  Fourier2 : Subsystem  mask(Fourier analyser){f1=Freq, n=0}
      mask prompts: f1 "Fundamental frequency f1 (Hz):"; n "Harmonic n (0=DC; 1=fundamental; 2=2nd harm;  ...) :"
      mask help: The Fourier block performs a Fourier analysis of the input signal over a running window of one cycle of the fundamental frequency. First and second outputs return respectively the magnitude and phase (degrees) of the harmonic component specified.
      mask init:
      | k=2-(n==0);
      mask Help: helpview(psbhelp)
  Math Function : Math  Operator=hypot  SaturateOnIntegerOverflow=on
  Terminator : Terminator
  Terminator1 : Terminator
  Out1 : Outport
  wires:
  Complex to Real-Imag/1 -> Fourier1/1(signal)
  Complex to Real-Imag/2 -> Fourier2/1(signal)
  Fourier1/2(angle) -> Terminator/1
  Fourier2/2(angle) -> Terminator1/1
  Fourier1/1(magnitude) -> Math Function/1
  Fourier2/1(magnitude) -> Math Function/2
  Math Function/1 -> Out1/1
  In1/1 -> Complex to Real-Imag/1

== system power_wind/Wind Farm/Wind Turbine Protections/Protection System1/AC Voltage Protection/Voltage Measurement/magnitude2 ==
  In1 : Inport
  Complex to Real-Imag : ComplexToRealImag
  Fourier1 : Subsystem  mask(Fourier analyser){f1=Freq, n=0}
      mask prompts: f1 "Fundamental frequency f1 (Hz):"; n "Harmonic n (0=DC; 1=fundamental; 2=2nd harm;  ...) :"
      mask help: The Fourier block performs a Fourier analysis of the input signal over a running window of one cycle of the fundamental frequency. First and second outputs return respectively the magnitude and phase (degrees) of the harmonic component specified.
      mask init:
      | k=2-(n==0);
      mask Help: helpview(psbhelp)
  Fourier2 : Subsystem  mask(Fourier analyser){f1=Freq, n=0}
      mask prompts: f1 "Fundamental frequency f1 (Hz):"; n "Harmonic n (0=DC; 1=fundamental; 2=2nd harm;  ...) :"
      mask help: The Fourier block performs a Fourier analysis of the input signal over a running window of one cycle of the fundamental frequency. First and second outputs return respectively the magnitude and phase (degrees) of the harmonic component specified.
      mask init:
      | k=2-(n==0);
      mask Help: helpview(psbhelp)
  Math Function : Math  Operator=hypot  SaturateOnIntegerOverflow=on
  Terminator : Terminator
  Terminator1 : Terminator
  Out1 : Outport
  wires:
  In1/1 -> Complex to Real-Imag/1
  Math Function/1 -> Out1/1
  Fourier2/1(magnitude) -> Math Function/2
  Fourier1/1(magnitude) -> Math Function/1
  Fourier2/2(angle) -> Terminator1/1
  Fourier1/2(angle) -> Terminator/1
  Complex to Real-Imag/2 -> Fourier2/1(signal)
  Complex to Real-Imag/1 -> Fourier1/1(signal)

== system power_wind/Wind Farm/Wind Turbine Protections/Protection System2/AC Current Protection/Current Measurement/magnitude ==
  In1 : Inport
  Complex to Real-Imag : ComplexToRealImag
  Fourier1 : Subsystem  mask(Fourier analyser){f1=Freq, n=0}
      mask prompts: f1 "Fundamental frequency f1 (Hz):"; n "Harmonic n (0=DC; 1=fundamental; 2=2nd harm;  ...) :"
      mask help: The Fourier block performs a Fourier analysis of the input signal over a running window of one cycle of the fundamental frequency. First and second outputs return respectively the magnitude and phase (degrees) of the harmonic component specified.
      mask init:
      | k=2-(n==0);
      mask Help: helpview(psbhelp)
  Fourier2 : Subsystem  mask(Fourier analyser){f1=Freq, n=0}
      mask prompts: f1 "Fundamental frequency f1 (Hz):"; n "Harmonic n (0=DC; 1=fundamental; 2=2nd harm;  ...) :"
      mask help: The Fourier block performs a Fourier analysis of the input signal over a running window of one cycle of the fundamental frequency. First and second outputs return respectively the magnitude and phase (degrees) of the harmonic component specified.
      mask init:
      | k=2-(n==0);
      mask Help: helpview(psbhelp)
  Math Function : Math  Operator=hypot  SaturateOnIntegerOverflow=on
  Terminator : Terminator
  Terminator1 : Terminator
  Out1 : Outport
  wires:
  Complex to Real-Imag/1 -> Fourier1/1(signal)
  Complex to Real-Imag/2 -> Fourier2/1(signal)
  Fourier1/2(angle) -> Terminator/1
  Fourier2/2(angle) -> Terminator1/1
  Fourier1/1(magnitude) -> Math Function/1
  Fourier2/1(magnitude) -> Math Function/2
  Math Function/1 -> Out1/1
  In1/1 -> Complex to Real-Imag/1

== system power_wind/Wind Farm/Wind Turbine Protections/Protection System2/AC Current Protection/Current Measurement/magnitude1 ==
  In1 : Inport
  Complex to Real-Imag : ComplexToRealImag
  Fourier1 : Subsystem  mask(Fourier analyser){f1=Freq, n=0}
      mask prompts: f1 "Fundamental frequency f1 (Hz):"; n "Harmonic n (0=DC; 1=fundamental; 2=2nd harm;  ...) :"
      mask help: The Fourier block performs a Fourier analysis of the input signal over a running window of one cycle of the fundamental frequency. First and second outputs return respectively the magnitude and phase (degrees) of the harmonic component specified.
      mask init:
      | k=2-(n==0);
      mask Help: helpview(psbhelp)
  Fourier2 : Subsystem  mask(Fourier analyser){f1=Freq, n=0}
      mask prompts: f1 "Fundamental frequency f1 (Hz):"; n "Harmonic n (0=DC; 1=fundamental; 2=2nd harm;  ...) :"
      mask help: The Fourier block performs a Fourier analysis of the input signal over a running window of one cycle of the fundamental frequency. First and second outputs return respectively the magnitude and phase (degrees) of the harmonic component specified.
      mask init:
      | k=2-(n==0);
      mask Help: helpview(psbhelp)
  Math Function : Math  Operator=hypot  SaturateOnIntegerOverflow=on
  Terminator : Terminator
  Terminator1 : Terminator
  Out1 : Outport
  wires:
  In1/1 -> Complex to Real-Imag/1
  Math Function/1 -> Out1/1
  Fourier2/1(magnitude) -> Math Function/2
  Fourier1/1(magnitude) -> Math Function/1
  Fourier2/2(angle) -> Terminator1/1
  Fourier1/2(angle) -> Terminator/1
  Complex to Real-Imag/2 -> Fourier2/1(signal)
  Complex to Real-Imag/1 -> Fourier1/1(signal)

== system power_wind/Wind Farm/Wind Turbine Protections/Protection System2/AC Voltage Protection/Voltage Measurement/magnitude ==
  In1 : Inport
  Complex to Real-Imag : ComplexToRealImag
  Fourier1 : Subsystem  mask(Fourier analyser){f1=Freq, n=0}
      mask prompts: f1 "Fundamental frequency f1 (Hz):"; n "Harmonic n (0=DC; 1=fundamental; 2=2nd harm;  ...) :"
      mask help: The Fourier block performs a Fourier analysis of the input signal over a running window of one cycle of the fundamental frequency. First and second outputs return respectively the magnitude and phase (degrees) of the harmonic component specified.
      mask init:
      | k=2-(n==0);
      mask Help: helpview(psbhelp)
  Fourier2 : Subsystem  mask(Fourier analyser){f1=Freq, n=0}
      mask prompts: f1 "Fundamental frequency f1 (Hz):"; n "Harmonic n (0=DC; 1=fundamental; 2=2nd harm;  ...) :"
      mask help: The Fourier block performs a Fourier analysis of the input signal over a running window of one cycle of the fundamental frequency. First and second outputs return respectively the magnitude and phase (degrees) of the harmonic component specified.
      mask init:
      | k=2-(n==0);
      mask Help: helpview(psbhelp)
  Math Function : Math  Operator=hypot  SaturateOnIntegerOverflow=on
  Terminator : Terminator
  Terminator1 : Terminator
  Out1 : Outport
  wires:
  Complex to Real-Imag/1 -> Fourier1/1(signal)
  Complex to Real-Imag/2 -> Fourier2/1(signal)
  Fourier1/2(angle) -> Terminator/1
  Fourier2/2(angle) -> Terminator1/1
  Fourier1/1(magnitude) -> Math Function/1
  Fourier2/1(magnitude) -> Math Function/2
  Math Function/1 -> Out1/1
  In1/1 -> Complex to Real-Imag/1

== system power_wind/Wind Farm/Wind Turbine Protections/Protection System2/AC Voltage Protection/Voltage Measurement/magnitude1 ==
  In1 : Inport
  Complex to Real-Imag : ComplexToRealImag
  Fourier1 : Subsystem  mask(Fourier analyser){f1=Freq, n=0}
      mask prompts: f1 "Fundamental frequency f1 (Hz):"; n "Harmonic n (0=DC; 1=fundamental; 2=2nd harm;  ...) :"
      mask help: The Fourier block performs a Fourier analysis of the input signal over a running window of one cycle of the fundamental frequency. First and second outputs return respectively the magnitude and phase (degrees) of the harmonic component specified.
      mask init:
      | k=2-(n==0);
      mask Help: helpview(psbhelp)
  Fourier2 : Subsystem  mask(Fourier analyser){f1=Freq, n=0}
      mask prompts: f1 "Fundamental frequency f1 (Hz):"; n "Harmonic n (0=DC; 1=fundamental; 2=2nd harm;  ...) :"
      mask help: The Fourier block performs a Fourier analysis of the input signal over a running window of one cycle of the fundamental frequency. First and second outputs return respectively the magnitude and phase (degrees) of the harmonic component specified.
      mask init:
      | k=2-(n==0);
      mask Help: helpview(psbhelp)
  Math Function : Math  Operator=hypot  SaturateOnIntegerOverflow=on
  Terminator : Terminator
  Terminator1 : Terminator
  Out1 : Outport
  wires:
  In1/1 -> Complex to Real-Imag/1
  Math Function/1 -> Out1/1
  Fourier2/1(magnitude) -> Math Function/2
  Fourier1/1(magnitude) -> Math Function/1
  Fourier2/2(angle) -> Terminator1/1
  Fourier1/2(angle) -> Terminator/1
  Complex to Real-Imag/2 -> Fourier2/1(signal)
  Complex to Real-Imag/1 -> Fourier1/1(signal)

== system power_wind/Wind Farm/Wind Turbine Protections/Protection System2/AC Voltage Protection/Voltage Measurement/magnitude2 ==
  In1 : Inport
  Complex to Real-Imag : ComplexToRealImag
  Fourier1 : Subsystem  mask(Fourier analyser){f1=Freq, n=0}
      mask prompts: f1 "Fundamental frequency f1 (Hz):"; n "Harmonic n (0=DC; 1=fundamental; 2=2nd harm;  ...) :"
      mask help: The Fourier block performs a Fourier analysis of the input signal over a running window of one cycle of the fundamental frequency. First and second outputs return respectively the magnitude and phase (degrees) of the harmonic component specified.
      mask init:
      | k=2-(n==0);
      mask Help: helpview(psbhelp)
  Fourier2 : Subsystem  mask(Fourier analyser){f1=Freq, n=0}
      mask prompts: f1 "Fundamental frequency f1 (Hz):"; n "Harmonic n (0=DC; 1=fundamental; 2=2nd harm;  ...) :"
      mask help: The Fourier block performs a Fourier analysis of the input signal over a running window of one cycle of the fundamental frequency. First and second outputs return respectively the magnitude and phase (degrees) of the harmonic component specified.
      mask init:
      | k=2-(n==0);
      mask Help: helpview(psbhelp)
  Math Function : Math  Operator=hypot  SaturateOnIntegerOverflow=on
  Terminator : Terminator
  Terminator1 : Terminator
  Out1 : Outport
  wires:
  Complex to Real-Imag/1 -> Fourier1/1(signal)
  Complex to Real-Imag/2 -> Fourier2/1(signal)
  Fourier1/2(angle) -> Terminator/1
  Fourier2/2(angle) -> Terminator1/1
  Fourier1/1(magnitude) -> Math Function/1
  Fourier2/1(magnitude) -> Math Function/2
  Math Function/1 -> Out1/1
  In1/1 -> Complex to Real-Imag/1

== system power_wind/Wind Farm/Wind Turbine Protections/Protection System3/AC Current Protection/Current Measurement/magnitude ==
  In1 : Inport
  Complex to Real-Imag : ComplexToRealImag
  Fourier1 : Subsystem  mask(Fourier analyser){f1=Freq, n=0}
      mask prompts: f1 "Fundamental frequency f1 (Hz):"; n "Harmonic n (0=DC; 1=fundamental; 2=2nd harm;  ...) :"
      mask help: The Fourier block performs a Fourier analysis of the input signal over a running window of one cycle of the fundamental frequency. First and second outputs return respectively the magnitude and phase (degrees) of the harmonic component specified.
      mask init:
      | k=2-(n==0);
      mask Help: helpview(psbhelp)
  Fourier2 : Subsystem  mask(Fourier analyser){f1=Freq, n=0}
      mask prompts: f1 "Fundamental frequency f1 (Hz):"; n "Harmonic n (0=DC; 1=fundamental; 2=2nd harm;  ...) :"
      mask help: The Fourier block performs a Fourier analysis of the input signal over a running window of one cycle of the fundamental frequency. First and second outputs return respectively the magnitude and phase (degrees) of the harmonic component specified.
      mask init:
      | k=2-(n==0);
      mask Help: helpview(psbhelp)
  Math Function : Math  Operator=hypot  SaturateOnIntegerOverflow=on
  Terminator : Terminator
  Terminator1 : Terminator
  Out1 : Outport
  wires:
  In1/1 -> Complex to Real-Imag/1
  Math Function/1 -> Out1/1
  Fourier2/1(magnitude) -> Math Function/2
  Fourier1/1(magnitude) -> Math Function/1
  Fourier2/2(angle) -> Terminator1/1
  Fourier1/2(angle) -> Terminator/1
  Complex to Real-Imag/2 -> Fourier2/1(signal)
  Complex to Real-Imag/1 -> Fourier1/1(signal)

== system power_wind/Wind Farm/Wind Turbine Protections/Protection System3/AC Current Protection/Current Measurement/magnitude1 ==
  In1 : Inport
  Complex to Real-Imag : ComplexToRealImag
  Fourier1 : Subsystem  mask(Fourier analyser){f1=Freq, n=0}
      mask prompts: f1 "Fundamental frequency f1 (Hz):"; n "Harmonic n (0=DC; 1=fundamental; 2=2nd harm;  ...) :"
      mask help: The Fourier block performs a Fourier analysis of the input signal over a running window of one cycle of the fundamental frequency. First and second outputs return respectively the magnitude and phase (degrees) of the harmonic component specified.
      mask init:
      | k=2-(n==0);
      mask Help: helpview(psbhelp)
  Fourier2 : Subsystem  mask(Fourier analyser){f1=Freq, n=0}
      mask prompts: f1 "Fundamental frequency f1 (Hz):"; n "Harmonic n (0=DC; 1=fundamental; 2=2nd harm;  ...) :"
      mask help: The Fourier block performs a Fourier analysis of the input signal over a running window of one cycle of the fundamental frequency. First and second outputs return respectively the magnitude and phase (degrees) of the harmonic component specified.
      mask init:
      | k=2-(n==0);
      mask Help: helpview(psbhelp)
  Math Function : Math  Operator=hypot  SaturateOnIntegerOverflow=on
  Terminator : Terminator
  Terminator1 : Terminator
  Out1 : Outport
  wires:
  Complex to Real-Imag/1 -> Fourier1/1(signal)
  Complex to Real-Imag/2 -> Fourier2/1(signal)
  Fourier1/2(angle) -> Terminator/1
  Fourier2/2(angle) -> Terminator1/1
  Fourier1/1(magnitude) -> Math Function/1
  Fourier2/1(magnitude) -> Math Function/2
  Math Function/1 -> Out1/1
  In1/1 -> Complex to Real-Imag/1

== system power_wind/Wind Farm/Wind Turbine Protections/Protection System3/AC Voltage Protection/Voltage Measurement/magnitude ==
  In1 : Inport
  Complex to Real-Imag : ComplexToRealImag
  Fourier1 : Subsystem  mask(Fourier analyser){f1=Freq, n=0}
      mask prompts: f1 "Fundamental frequency f1 (Hz):"; n "Harmonic n (0=DC; 1=fundamental; 2=2nd harm;  ...) :"
      mask help: The Fourier block performs a Fourier analysis of the input signal over a running window of one cycle of the fundamental frequency. First and second outputs return respectively the magnitude and phase (degrees) of the harmonic component specified.
      mask init:
      | k=2-(n==0);
      mask Help: helpview(psbhelp)
  Fourier2 : Subsystem  mask(Fourier analyser){f1=Freq, n=0}
      mask prompts: f1 "Fundamental frequency f1 (Hz):"; n "Harmonic n (0=DC; 1=fundamental; 2=2nd harm;  ...) :"
      mask help: The Fourier block performs a Fourier analysis of the input signal over a running window of one cycle of the fundamental frequency. First and second outputs return respectively the magnitude and phase (degrees) of the harmonic component specified.
      mask init:
      | k=2-(n==0);
      mask Help: helpview(psbhelp)
  Math Function : Math  Operator=hypot  SaturateOnIntegerOverflow=on
  Terminator : Terminator
  Terminator1 : Terminator
  Out1 : Outport
  wires:
  In1/1 -> Complex to Real-Imag/1
  Math Function/1 -> Out1/1
  Fourier2/1(magnitude) -> Math Function/2
  Fourier1/1(magnitude) -> Math Function/1
  Fourier2/2(angle) -> Terminator1/1
  Fourier1/2(angle) -> Terminator/1
  Complex to Real-Imag/2 -> Fourier2/1(signal)
  Complex to Real-Imag/1 -> Fourier1/1(signal)
